simulink model "IT2_FPID_Controller"  (R2018b)
settings: Solver=ode4  StartTime=0.0  StopTime=8  FixedStep=0.05  RelTol=1e-3  EnableMultiTasking=on
values from neighbouring files (symbols this model uses):
  K = 1.8    [runControlSystemExample.m]
  Ka = 0.0002/6    (= 3.33333333333e-05)    [runControlSystemExample.m]
  Kb = 4    [runControlSystemExample.m]
  Kd = 0.01/6    (= 0.00166666666667)    [runControlSystemExample.m]
  Ke = 5.2    [runControlSystemExample.m]
  L = 0.1    [runControlSystemExample.m]
  T = 0.1    [runControlSystemExample.m]
undefined symbols (not defined in the file or in its folder): evalt2
settings Model: Creator=u11f99  LastModifiedBy=Ivan Milin
settings DataIOCC: LimitDataPoints=on  SaveFormat=Array
settings OptimizationCC: ExpressionDepthLimit=2147483647  LifeSpan=inf
settings DebuggingCC: UnderspecifiedInitializationDetection=Classic  MergeDetectMultiDrivingBlocksExec=none  SolverPrmCheckMsg=warning  AllowSymbolicDim=off  StateNameClashWarn=warning  SFUnexpectedBacktrackingDiag=warning  SFNoUnconditionalDefaultTransitionDiag=warning  SFExecutionAtInitializationDiag=none
settings HardwareCC: ProdBitPerPointer=32  ProdBitPerSizeT=32  ProdBitPerPtrDiffT=32  ProdLargestAtomicFloat=None  ProdIntDivRoundTo=Undefined  ProdEndianess=Unspecified  ProdWordSize=32  ProdHWDeviceType=32-bit Generic
settings ModelReferenceCC: PropagateSignalLabelsOutOfModel=off
settings SFSimCC: SimUseLocalCustomCode=off
settings RTWCC: RTWUseLocalCustomCode=off
settings CodeAppCC: StateflowObjectComments=on
settings GRTTargetCC: TargetLangStandard=C89/C90 (ANSI)  GeneratePreprocessorConditionals=Disable all
settings ConfigComp: CovMetricSettings=dw  CovHtmlReporting=on  CovSaveCumulativeToWorkspaceVar=on  CovSaveSingleToWorkspaceVar=on  CovExternalEMLEnable=off

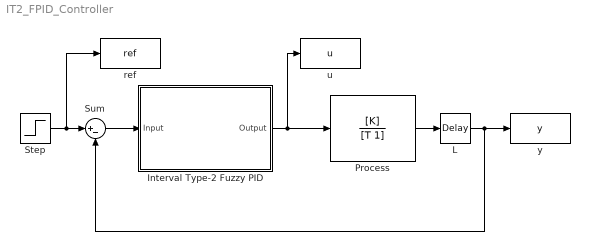
== system IT2_FPID_Controller ==
  Interval Type-2 Fuzzy PID : Subsystem
  L : TransportDelay  DelayTime=L
  Process : TransferFcn  Numerator=[K]  Denominator=[T 1]
  Step : Step  SampleTime=0
  Sum : Sum  Inputs=|+-
  ref : ToWorkspace  VariableName=ref  SaveFormat=Structure With Time  SampleTime=-1
  u : ToWorkspace  VariableName=u  SaveFormat=Structure With Time  SampleTime=-1
  y : ToWorkspace  VariableName=y  SaveFormat=Structure With Time  SampleTime=-1
  wires:
  Step/1 -> ref/1, Sum/1
  Sum/1 -> Interval Type-2 Fuzzy PID/1(Input)
  Process/1 -> L/1
  L/1 -> Sum/2, y/1
  Interval Type-2 Fuzzy PID/1(Output) -> u/1, Process/1

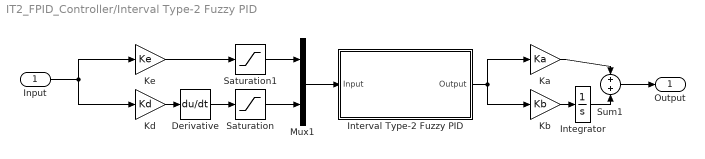
== system IT2_FPID_Controller/Interval Type-2 Fuzzy PID ==
  Input : Inport
  Derivative : Derivative
  Integrator : Integrator
  Interval Type-2 Fuzzy PID : Subsystem  AncestorBlock=Fuzzy_Type2_Lib/Interval Type-2 Fuzzy Logic Controller with TR selection  mask(Type-2 Fuzzy Logic Controller){t2fisSim=t2fisSim, TRtype=7}
      mask prompts: t2fisSim "t2fis name in Workspace or File Name"; TRtype "Select TR method"
      mask help:
      | TR Method List for selection;
      |
      | 1 - Karnik-Mendel Algorithm (KM)
      | 2 - Enhanced Karnik-Mendel Algorithm(EKM)
      | 3 - Iterative Algorithm with Stop Condition(IASC)
      | 4 - Enhanced Iterative Algorithm with Stop Condition(EIASC)
      | 5 - Enhanced Opposite Direction Searching Algorithm(EODS)
      | 6 - wu-Mendel Uncertainity Bound Method(WM)
      | 7 - Nie-Tan Method(NT)
      | 8 - Begain-Melek-Mendel Method(BMM)
      | 9 - User Defined Function
      mask Display: image(imread('MemberShipMask.jpg'))
  Ka : Gain  Gain=Ka
  Kb : Gain  Gain=Kb
  Kd : Gain  Gain=Kd
  Ke : Gain  Gain=Ke
  Mux1 : Mux  Inputs=2
  Saturation : Saturate  UpperLimit=1  LowerLimit=-1
  Saturation1 : Saturate  UpperLimit=1  LowerLimit=-1
  Sum1 : Sum
  Output : Outport
  wires:
  Saturation1/1 -> Mux1/1
  Saturation/1 -> Mux1/2
  Derivative/1 -> Saturation/1
  Kd/1 -> Derivative/1
  Ke/1 -> Saturation1/1
  Input/1 -> Kd/1, Ke/1
  Interval Type-2 Fuzzy PID/1(Output) -> Kb/1, Ka/1
  Kb/1 -> Integrator/1
  Integrator/1 -> Sum1/2
  Ka/1 -> Sum1/1
  Sum1/1 -> Output/1
  Mux1/1 -> Interval Type-2 Fuzzy PID/1(Input)

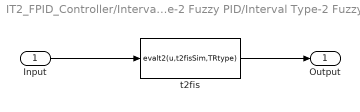
== system IT2_FPID_Controller/Interval Type-2 Fuzzy PID/Interval Type-2 Fuzzy PID ==
  Input : Inport
  t2fis : MATLABFcn  MATLABFcn=evalt2(u,t2fisSim,TRtype)  OutputDimensions=1
  Output : Outport
  wires:
  Input/1 -> t2fis/1
  t2fis/1 -> Output/1
